simulink model "hrtf_filter"  (R2025a)
settings: Solver=FixedStepDiscrete  StartTime=0.0  StopTime=10.0  FixedStep=1/48000  RelTol=1e-3
undefined symbols (not defined in the file): channel, dspblkCoreblockFVToolHelper, gcbh, HRIR
settings Model: Creator=eoencue1  LastModifiedBy=eoencue1
settings OptimizationCC: DefaultParameterBehavior=Inlined  EnhancedBackFolding=on  PassReuseOutputArgsAs=Individual arguments  OptimizeBlockOrder=speed  DifferentSizesBufferReuse=on  OptimizationCustomize=off  EfficientTunableParamExpr=on
settings DebuggingCC: SignalRangeChecking=warning  ParameterTunabilityLossMsg=error
settings HardwareCC: ProdBitPerPointer=32.0  ProdBitPerSizeT=32.0  ProdBitPerPtrDiffT=32.0  ProdLargestAtomicFloat=None  ProdWordSize=32.0  ProdLongLongMode=on  ProdHWDeviceType=Custom Processor->Custom Processor
settings SFSimCC: MATLABDynamicMemAlloc=off
settings RTWCC: SystemTargetFile=ert.tlc  GenCodeOnly=on  TemplateMakefile=ert_default_tmf  Description=Embedded Coder
settings CodeAppCC: ForceParamTrailComments=on  IgnoreCustomStorageClasses=off  OperatorAnnotations=on  SimulinkDataObjDesc=on  SFDataObjDesc=on  InsertBlockDesc=on
settings ERTTargetCC: ExtModeTransport=0.0  ExtModeStaticAlloc=off  ExtModeMexFile=ext_comm  ExtModeIntrfLevel=Level1  ERTCustomFileTemplate=example_file_process.tlc  TargetLangStandard=C99 (ISO)  GenerateSampleERTMain=on  CodeInterfacePackaging=Reusable function  SupportNonFinite=off

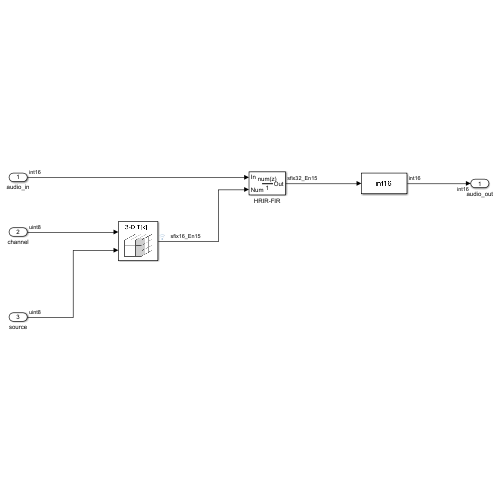
[thumbnail: Simulink's stored preview of the top-level diagram]
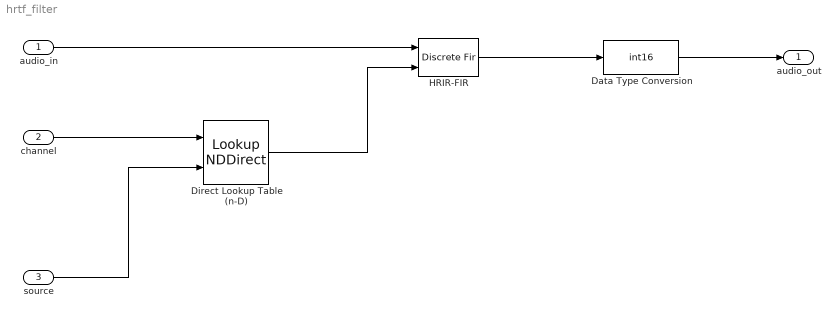
== system hrtf_filter ==
  audio_in : Inport  OutMin=-32768  OutMax=32767  OutDataTypeStr=int16  PortDimensions=1
  channel : Inport  Port=2  OutDataTypeStr=uint8
  source : Inport  Port=3  OutDataTypeStr=uint8
  Data Type Conversion : DataTypeConversion  OutDataTypeStr=int16  RndMeth=Floor
  Direct Lookup Table (n-D) : LookupNDDirect  NumberOfTableDimensions=3  InputsSelectThisObjectFromTable=Vector  Table=HRIR  TableDataTypeStr=fixdt(1,16,15)
  HRIR-FIR : DiscreteFir  LoadFcn=dspblkCoreblockFVToolHelper(gcbh,'load');  CoefSource=Input port  Coefficients=HRIR(channel,:)  CoefDataTypeStr=fixdt(1,16,15)  ProductDataTypeStr=fixdt(1,32,15)  AccumDataTypeStr=fixdt(1,32,15)
      settings: CopyFcn=dspblkCoreblockFVToolHelper(gcbh,'copy');  DeleteFcn=dspblkCoreblockFVToolHelper(gcbh,'close');  ModelCloseFcn=dspblkCoreblockFVToolHelper(gcbh,'close');  PreSaveFcn=dspblkCoreblockFVToolHelper(gcbh,'presave');  PostSaveFcn=dspblkCoreblockFVToolHelper(gcbh,'postsave');  CloseFcn=dspblkCoreblockFVToolHelper(gcbh,'close');  InputPortMap=u0,u1
  audio_out : Outport  OutDataTypeStr=int16
  wires:
  audio_in/1 -> HRIR-FIR/1
  HRIR-FIR/1 -> Data Type Conversion/1
  channel/1 -> Direct Lookup Table (n-D)/1
  Direct Lookup Table (n-D)/1 -> HRIR-FIR/2
  Data Type Conversion/1 -> audio_out/1
  source/1 -> Direct Lookup Table (n-D)/2
